simulink model "S215"  (R2024b)
settings: Solver=FixedStepAuto  StartTime=0.0  StopTime=0.1  FixedStep=1e-6  RelTol=1e-3
libraries: simulink x1
settings Model: Creator=86195  LastModifiedBy=86195

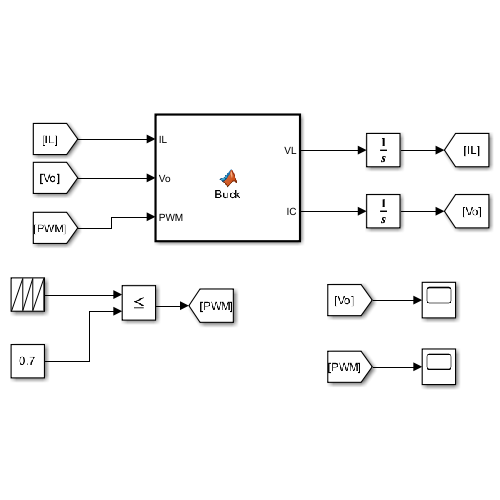
[thumbnail: Simulink's stored preview of the top-level diagram]
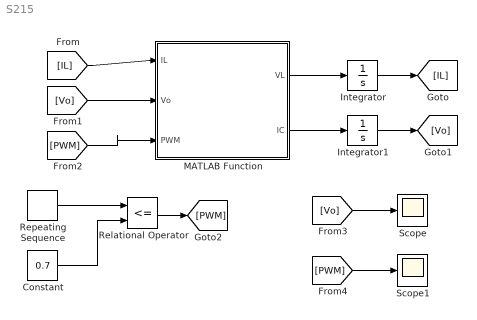
== system S215 ==
  Constant : Constant  Value=0.7
  Integrator : Integrator
  Integrator1 : Integrator
  MATLAB Function : MATLAB Function  TreatAsAtomicUnit=on
  Relational Operator : RelationalOperator  Operator=<=  OutDataTypeStr=boolean  RndMeth=Simplest  InputSameDT=off
  Repeating Sequence : simulink/Sources/Repeating Sequence  rep_seq_t=[0 1e-4]  rep_seq_y=[0 1]
  Scope : Scope
  Scope1 : Scope
  wires:
  MATLAB Function/1(VL) -> Integrator/1
  MATLAB Function/2(IC) -> Integrator1/1
  Integrator/1 -> [IL]
  Integrator1/1 -> [Vo]
  [IL] -> MATLAB Function/1(IL)
  [Vo] -> MATLAB Function/2(Vo)
  Relational Operator/1 -> [PWM]
  [PWM] -> MATLAB Function/3(PWM)
  Repeating Sequence/1 -> Relational Operator/1
  Constant/1 -> Relational Operator/2
  [Vo] -> Scope/1
  [PWM] -> Scope1/1

== matlab function S215/MATLAB Function ==
  data: IL input; VL output; Vo input; PWM input; IC output
function [VL,IC]= Buck(IL, Vo, PWM)
%% 参 数
Vg = 100;
L = 1e-3;
C = 470e-6;
R = 10;
Io = Vo/R;
if (PWM > 0)
%% 电 感 电 压、 电 容 电 流 公 式
VL = (Vg - Vo)/L;
else
VL = -Vo/L;
end
IC = (IL - Io)/C;
